simulink model "packetizer_core"  (R2016b)
settings: Solver=VariableStepAuto  StartTime=0.0  StopTime=2*64*512+100  RelTol=1e-3
model workspace (MAT data in the model file):
  dstin = [0 168430081 168430082 168430083 168430084 168430085 168430086 168430087 168430088 168430089 168430090 168430091 ... (33 elements, 1x33)]
  simin = [1 2 3 4 5 6 7 8 9 10 11 12 ... (262544 elements, 65636x4)]
libraries: xbsIndex_r4 x142
(part 2 of 2)

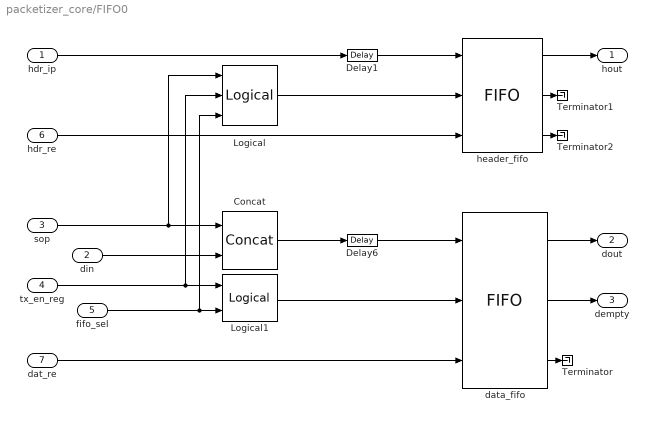
== system packetizer_core/FIFO0 ==
  hdr_ip : Inport
  din : Inport  Port=2
  sop : Inport  Port=3
  tx_en_reg : Inport  Port=4
  fifo_sel : Inport  Port=5
  hdr_re : Inport  Port=6
  dat_re : Inport  Port=7
  Concat : xbsIndex_r4/Concat  num_inputs=2  dbl_ovrd=off  block_type=concat
  Delay1 : xbsIndex_r4/Delay  rst=off  infoeditControl=Selection of Reset will increase slice count due to use of real FFs and instead of SRLs  en=off  latency=1  reg_retiming=off  dbl_ovrd=off  block_type=delay
  Delay6 : xbsIndex_r4/Delay  rst=off  infoeditControl=Selection of Reset will increase slice count due to use of real FFs and instead of SRLs  en=off  latency=1  reg_retiming=off  dbl_ovrd=off  block_type=delay
  Logical : xbsIndex_r4/Logical  logical_function=AND  inputs=3  en=off  latency=1  precision=Full  arith_type=Unsigned  n_bits=16  bin_pt=0  align_bp=on  dbl_ovrd=off  block_type=logical
  Logical1 : xbsIndex_r4/Logical  logical_function=AND  inputs=2  en=off  latency=1  precision=Full  arith_type=Unsigned  n_bits=16  bin_pt=0  align_bp=on  dbl_ovrd=off  block_type=logical
  Terminator : Terminator
  Terminator1 : Terminator
  Terminator2 : Terminator
  data_fifo : xbsIndex_r4/FIFO  mem_type=Block RAM  performance_options=First_Word_Fall_Through  embedded_registers=on  depth=16K  percent_nbits=1  rst=off  rst_latency=1  en=off  use_dcount=off  use_percent_full_port=off  use_almost_empty=off  almost_empty_thresh=2  use_almost_full=off  almost_full_thresh=14  explicit_period=off  dbl_ovrd=off  block_type=fifo
  header_fifo : xbsIndex_r4/FIFO  mem_type=Distributed RAM  performance_options=First_Word_Fall_Through  embedded_registers=off  depth=32  percent_nbits=1  rst=off  rst_latency=1  en=off  use_dcount=off  use_percent_full_port=off  use_almost_empty=off  almost_empty_thresh=2  use_almost_full=off  almost_full_thresh=14  explicit_period=off  dbl_ovrd=off  block_type=fifo
  hout : Outport
  dout : Outport  Port=2
  dempty : Outport  Port=3
  wires:
  Logical/1 -> header_fifo/2
  tx_en_reg/1 -> Logical1/1, Logical/2
  Delay1/1 -> header_fifo/1
  Delay6/1 -> data_fifo/1
  data_fifo/1 -> dout/1
  data_fifo/2 -> dempty/1
  Logical1/1 -> data_fifo/2
  dat_re/1 -> data_fifo/3
  hdr_re/1 -> header_fifo/3
  hdr_ip/1 -> Delay1/1
  Concat/1 -> Delay6/1
  header_fifo/1 -> hout/1
  sop/1 -> Concat/1, Logical/1
  din/1 -> Concat/2
  fifo_sel/1 -> Logical1/2, Logical/3
  data_fifo/3 -> Terminator/1
  header_fifo/2 -> Terminator1/1
  header_fifo/3 -> Terminator2/1

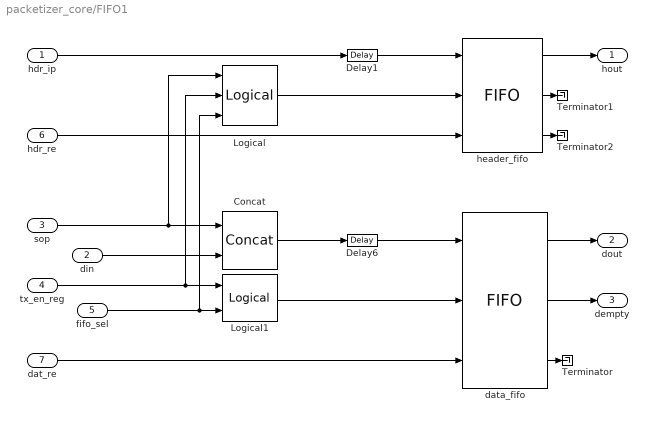
== system packetizer_core/FIFO1 ==
  hdr_ip : Inport
  din : Inport  Port=2
  sop : Inport  Port=3
  tx_en_reg : Inport  Port=4
  fifo_sel : Inport  Port=5
  hdr_re : Inport  Port=6
  dat_re : Inport  Port=7
  Concat : xbsIndex_r4/Concat  num_inputs=2  dbl_ovrd=off  block_type=concat
  Delay1 : xbsIndex_r4/Delay  rst=off  infoeditControl=Selection of Reset will increase slice count due to use of real FFs and instead of SRLs  en=off  latency=1  reg_retiming=off  dbl_ovrd=off  block_type=delay
  Delay6 : xbsIndex_r4/Delay  rst=off  infoeditControl=Selection of Reset will increase slice count due to use of real FFs and instead of SRLs  en=off  latency=1  reg_retiming=off  dbl_ovrd=off  block_type=delay
  Logical : xbsIndex_r4/Logical  logical_function=AND  inputs=3  en=off  latency=1  precision=Full  arith_type=Unsigned  n_bits=16  bin_pt=0  align_bp=on  dbl_ovrd=off  block_type=logical
  Logical1 : xbsIndex_r4/Logical  logical_function=AND  inputs=2  en=off  latency=1  precision=Full  arith_type=Unsigned  n_bits=16  bin_pt=0  align_bp=on  dbl_ovrd=off  block_type=logical
  Terminator : Terminator
  Terminator1 : Terminator
  Terminator2 : Terminator
  data_fifo : xbsIndex_r4/FIFO  mem_type=Block RAM  performance_options=First_Word_Fall_Through  embedded_registers=on  depth=16K  percent_nbits=1  rst=off  rst_latency=1  en=off  use_dcount=off  use_percent_full_port=off  use_almost_empty=off  almost_empty_thresh=2  use_almost_full=off  almost_full_thresh=14  explicit_period=off  dbl_ovrd=off  block_type=fifo
  header_fifo : xbsIndex_r4/FIFO  mem_type=Distributed RAM  performance_options=First_Word_Fall_Through  embedded_registers=off  depth=32  percent_nbits=1  rst=off  rst_latency=1  en=off  use_dcount=off  use_percent_full_port=off  use_almost_empty=off  almost_empty_thresh=2  use_almost_full=off  almost_full_thresh=14  explicit_period=off  dbl_ovrd=off  block_type=fifo
  hout : Outport
  dout : Outport  Port=2
  dempty : Outport  Port=3
  wires:
  Logical/1 -> header_fifo/2
  tx_en_reg/1 -> Logical1/1, Logical/2
  Delay1/1 -> header_fifo/1
  Delay6/1 -> data_fifo/1
  data_fifo/1 -> dout/1
  data_fifo/2 -> dempty/1
  Logical1/1 -> data_fifo/2
  dat_re/1 -> data_fifo/3
  hdr_re/1 -> header_fifo/3
  hdr_ip/1 -> Delay1/1
  Concat/1 -> Delay6/1
  header_fifo/1 -> hout/1
  sop/1 -> Concat/1, Logical/1
  din/1 -> Concat/2
  fifo_sel/1 -> Logical1/2, Logical/3
  data_fifo/3 -> Terminator/1
  header_fifo/2 -> Terminator1/1
  header_fifo/3 -> Terminator2/1

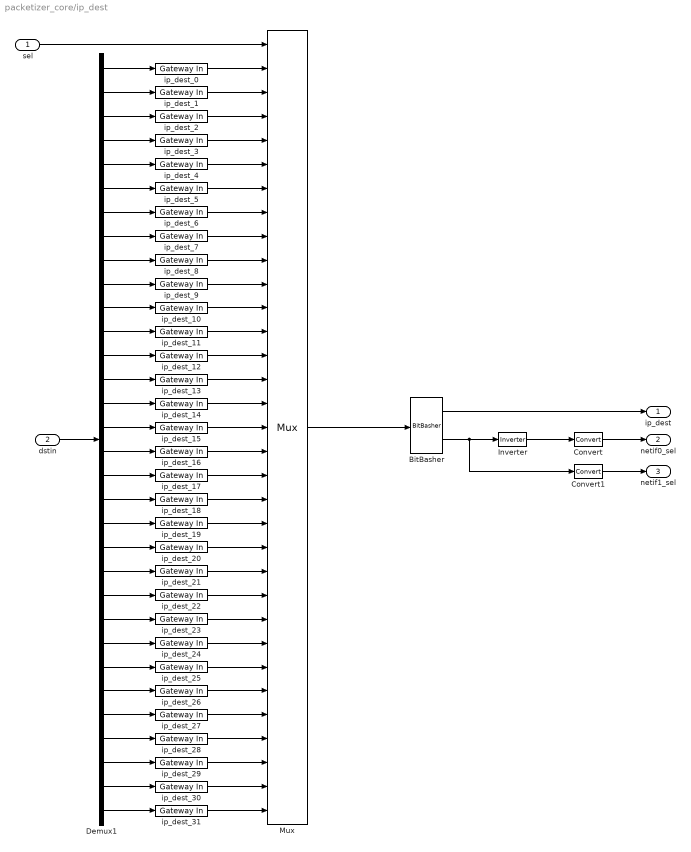
== system packetizer_core/ip_dest ==
  sel : Inport
  dstin : Inport  Port=2
  BitBasher : xbsIndex_r4/BitBasher  bitexpr=|  display_expr=off  sr_1=ip  arith_type1=Unsigned  bin_pt1=0  sr_2=sel  arith_type2=Unsigned  bin_pt2=0  sr_3=3  arith_type3=Unsigned  bin_pt3=0  sr_4=4  arith_type4=Unsigned  bin_pt4=0  dbl_ovrd=off  block_type=bitbasher
      | ip={in[31:25], 1'b0, in[23:0]}
      | sel={in[24]}
  Convert : xbsIndex_r4/Convert  gui_display_data_type=Boolean  arith_type=Boolean  n_bits=16  bin_pt=14  float_type=Single  exp_bits=8  fraction_bits=24  quantization=Truncate  overflow=Wrap  en=off  latency=0  pipeline=off  dbl_ovrd=off  block_type=convert
  Convert1 : xbsIndex_r4/Convert  gui_display_data_type=Boolean  arith_type=Boolean  n_bits=16  bin_pt=14  float_type=Single  exp_bits=8  fraction_bits=24  quantization=Truncate  overflow=Wrap  en=off  latency=0  pipeline=off  dbl_ovrd=off  block_type=convert
  Demux1 : Demux  Outputs=32
  Inverter : xbsIndex_r4/Inverter  en=off  latency=0  dbl_ovrd=off  block_type=inv
  Mux : xbsIndex_r4/Mux  inputs=32  en=off  latency=1  precision=Full  arith_type=Unsigned  n_bits=16  bin_pt=14  quantization=Truncate  overflow=Wrap  dbl_ovrd=off  block_type=mux
  ip_dest_{0..31} (32 alike) : xbsIndex_r4/Gateway In  gui_display_data_type=Fixed-point  arith_type=Unsigned  n_bits=32  bin_pt=0  preci_type=Single  exp_width=8  frac_width=24  rows=1  columns=1  quantization="Round  (unbiased: +/- Inf)"  overflow=Saturate  period=1  UseAsADC=off  ADCChannel='1'  interface=None  automatic_assignment=on  address_offset=hex2dec('00')  intf_name=''  intf_description=''  default_value=0  timing_constraint=None  locs_specified=off  LOCs={}  io_standard={}  inherit_from_input=off  hdl_port=on  dbl_ovrd=off  block_type=gatewayin
  ip_dest : Outport
  netif0_sel : Outport  Port=2
  netif1_sel : Outport  Port=3
  wires:
  ip_dest_6/1 -> Mux/8
  Demux1/16 -> ip_dest_15/1
  ip_dest_25/1 -> Mux/27
  Demux1/14 -> ip_dest_13/1
  ip_dest_3/1 -> Mux/5
  Demux1/26 -> ip_dest_25/1
  Demux1/18 -> ip_dest_17/1
  Demux1/32 -> ip_dest_31/1
  Demux1/4 -> ip_dest_3/1
  ip_dest_26/1 -> Mux/28
  ip_dest_23/1 -> Mux/25
  Demux1/10 -> ip_dest_9/1
  Demux1/7 -> ip_dest_6/1
  ip_dest_4/1 -> Mux/6
  ip_dest_8/1 -> Mux/10
  ip_dest_0/1 -> Mux/2
  ip_dest_13/1 -> Mux/15
  ip_dest_16/1 -> Mux/18
  ip_dest_12/1 -> Mux/14
  ip_dest_28/1 -> Mux/30
  ip_dest_7/1 -> Mux/9
  ip_dest_15/1 -> Mux/17
  Demux1/25 -> ip_dest_24/1
  Demux1/19 -> ip_dest_18/1
  Demux1/29 -> ip_dest_28/1
  ip_dest_2/1 -> Mux/4
  ip_dest_5/1 -> Mux/7
  Demux1/8 -> ip_dest_7/1
  Demux1/6 -> ip_dest_5/1
  Demux1/17 -> ip_dest_16/1
  Demux1/15 -> ip_dest_14/1
  Demux1/2 -> ip_dest_1/1
  ip_dest_11/1 -> Mux/13
  ip_dest_20/1 -> Mux/22
  ip_dest_1/1 -> Mux/3
  ip_dest_14/1 -> Mux/16
  Demux1/30 -> ip_dest_29/1
  Demux1/23 -> ip_dest_22/1
  Demux1/21 -> ip_dest_20/1
  Demux1/28 -> ip_dest_27/1
  ip_dest_21/1 -> Mux/23
  Demux1/27 -> ip_dest_26/1
  Demux1/11 -> ip_dest_10/1
  ip_dest_18/1 -> Mux/20
  ip_dest_10/1 -> Mux/12
  ip_dest_27/1 -> Mux/29
  Demux1/1 -> ip_dest_0/1
  Demux1/5 -> ip_dest_4/1
  Demux1/24 -> ip_dest_23/1
  ip_dest_30/1 -> Mux/32
  Demux1/3 -> ip_dest_2/1
  ip_dest_24/1 -> Mux/26
  Demux1/9 -> ip_dest_8/1
  sel/1 -> Mux/1
  dstin/1 -> Demux1/1
  Demux1/12 -> ip_dest_11/1
  ip_dest_17/1 -> Mux/19
  Demux1/20 -> ip_dest_19/1
  ip_dest_31/1 -> Mux/33
  Demux1/13 -> ip_dest_12/1
  ip_dest_19/1 -> Mux/21
  ip_dest_29/1 -> Mux/31
  ip_dest_22/1 -> Mux/24
  ip_dest_9/1 -> Mux/11
  Demux1/22 -> ip_dest_21/1
  Demux1/31 -> ip_dest_30/1
  Mux/1 -> BitBasher/1
  BitBasher/1 -> ip_dest/1
  BitBasher/2 -> Convert1/1, Inverter/1
  Inverter/1 -> Convert/1
  Convert/1 -> netif0_sel/1
  Convert1/1 -> netif1_sel/1

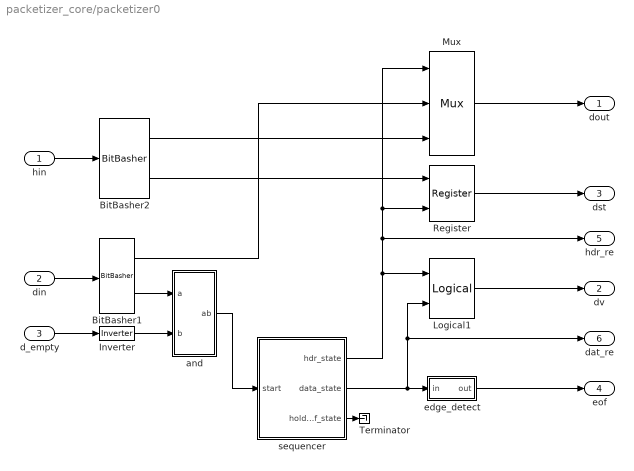
== system packetizer_core/packetizer0 ==
  hin : Inport
  din : Inport  Port=2
  d_empty : Inport  Port=3
  BitBasher1 : xbsIndex_r4/BitBasher  bitexpr=|  display_expr=off  sr_1=d  arith_type1=Unsigned  bin_pt1=0  sr_2=s  arith_type2=Unsigned  bin_pt2=0  sr_3=3  arith_type3=Unsigned  bin_pt3=0  sr_4=4  arith_type4=Unsigned  bin_pt4=0  dbl_ovrd=off  block_type=bitbasher
      | d={sd[63:0]}
      | s={sd[64]}
  BitBasher2 : xbsIndex_r4/BitBasher  bitexpr=|  display_expr=off  sr_1=hdr  arith_type1=Unsigned  bin_pt1=0  sr_2=ip  arith_type2=Unsigned  bin_pt2=0  sr_3=3  arith_type3=Unsigned  bin_pt3=0  sr_4=4  arith_type4=Unsigned  bin_pt4=0  dbl_ovrd=off  block_type=bitbasher
      | hdr={hdr_ip[95:32]}
      | ip={hdr_ip[31:0]}
  Inverter : xbsIndex_r4/Inverter  en=off  latency=0  dbl_ovrd=off  block_type=inv
  Logical1 : xbsIndex_r4/Logical  logical_function=OR  inputs=2  en=off  latency=1  precision=Full  arith_type=Unsigned  n_bits=16  bin_pt=0  align_bp=on  dbl_ovrd=off  block_type=logical
  Mux : xbsIndex_r4/Mux  inputs=2  en=off  latency=1  precision=Full  arith_type=Unsigned  n_bits=16  bin_pt=14  quantization=Truncate  overflow=Wrap  dbl_ovrd=off  block_type=mux
  Register : xbsIndex_r4/Register  init=0  rst=off  en=on  dbl_ovrd=off  block_type=register
  Terminator : Terminator
  and : Subsystem
  edge_detect : Subsystem  AncestorBlock=casper_library_misc/edge_detect  mask(edge_detect){edge=Falling, polarity=Active High, x_in=[0 0.08 0.08 0.16 0.16 0.24 0.24 0.32 0.32 0.4], y_in=[-1 -1  1  1  1  1  1  1  1  1], x_out=[0.6 0.68 0.68 0.76 0.76 0.84 0.84 0.92 0.92 1], y_out=[-1 -1  1  1 -1 -1 -1 -1 -1 -1]}
      mask prompts: edge "Edge Type"; polarity "Output Polarity"; x_in "Input X Positions"; y_in "Input Y Positions"; x_out "Output X Positions"; y_out "Output Y Positions"
      mask help: Output is active for one-cycle after each edge of the specified type (i.e. rising, falling or both).
      mask init:
      | edge_detect_init(gcb,...
      |     'edge',edge,...
      |     'polarity',polarity,...
      |     'x_in',x_in,...
      |     'x_out',x_out,...
      |     'y_in',y_in,...
      |     'y_out',y_out);
      | 
      | x_in_num=str2num(getfield(getfield(get_param(gcb,'UserData'),'parameters'),'x_in'));
      | x_out_num=str2num(getfield(getfield(get_param(gcb,'UserData'),'parameters'),'x_out'));
      | y_in_num=str2num(getfield(getfield(get_param(gcb,'UserData'),'parameters'),'y_in'));
      | y_out_num=str2num(getfield(getfield(get_param(gcb,'UserData'),'parameters'),'y_out'));
      settings: AttributesFormatString=|
      | falling edges
      | active high
      mask Help: Output is active for one-cycle after each edge of the specified type (i.e. rising, falling, or both).  Latency is zero.
      mask TypeOptions edge: Rising | Falling | Both
      mask TypeOptions polarity: Active High | Active Low
      mask Display:
      | plot(x_in_num,0.5+y_in_num*0.2);
      | plot(x_out_num,0.5+y_out_num*0.2);
  sequencer : Subsystem
  dout : Outport
  dv : Outport  Port=2
  dst : Outport  Port=3
  eof : Outport  Port=4
  hdr_re : Outport  Port=5
  dat_re : Outport  Port=6
  wires:
  din/1 -> BitBasher1/1
  d_empty/1 -> Inverter/1
  sequencer/1(hdr_state) -> Register/2, Mux/1, hdr_re/1, Logical1/1
  BitBasher1/1 -> Mux/2
  Mux/1 -> dout/1
  hin/1 -> BitBasher2/1
  BitBasher2/1 -> Mux/3
  Register/1 -> dst/1
  BitBasher2/2 -> Register/1
  sequencer/2(data_state) -> dat_re/1, Logical1/2, edge_detect/1(in)
  edge_detect/1(out) -> eof/1
  Logical1/1 -> dv/1
  sequencer/3(holdoff_state) -> Terminator/1
  BitBasher1/2 -> and/1(a)
  Inverter/1 -> and/2(b)
  and/1(ab) -> sequencer/1(start)

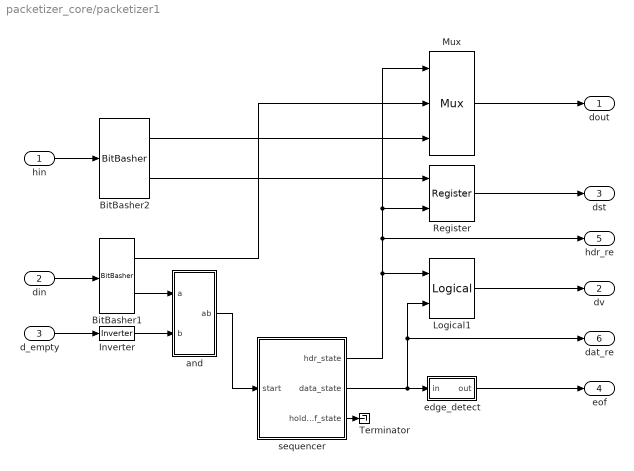
== system packetizer_core/packetizer1 ==
  hin : Inport
  din : Inport  Port=2
  d_empty : Inport  Port=3
  BitBasher1 : xbsIndex_r4/BitBasher  bitexpr=|  display_expr=off  sr_1=d  arith_type1=Unsigned  bin_pt1=0  sr_2=s  arith_type2=Unsigned  bin_pt2=0  sr_3=3  arith_type3=Unsigned  bin_pt3=0  sr_4=4  arith_type4=Unsigned  bin_pt4=0  dbl_ovrd=off  block_type=bitbasher
      | d={sd[63:0]}
      | s={sd[64]}
  BitBasher2 : xbsIndex_r4/BitBasher  bitexpr=|  display_expr=off  sr_1=hdr  arith_type1=Unsigned  bin_pt1=0  sr_2=ip  arith_type2=Unsigned  bin_pt2=0  sr_3=3  arith_type3=Unsigned  bin_pt3=0  sr_4=4  arith_type4=Unsigned  bin_pt4=0  dbl_ovrd=off  block_type=bitbasher
      | hdr={hdr_ip[95:32]}
      | ip={hdr_ip[31:0]}
  Inverter : xbsIndex_r4/Inverter  en=off  latency=0  dbl_ovrd=off  block_type=inv
  Logical1 : xbsIndex_r4/Logical  logical_function=OR  inputs=2  en=off  latency=1  precision=Full  arith_type=Unsigned  n_bits=16  bin_pt=0  align_bp=on  dbl_ovrd=off  block_type=logical
  Mux : xbsIndex_r4/Mux  inputs=2  en=off  latency=1  precision=Full  arith_type=Unsigned  n_bits=16  bin_pt=14  quantization=Truncate  overflow=Wrap  dbl_ovrd=off  block_type=mux
  Register : xbsIndex_r4/Register  init=0  rst=off  en=on  dbl_ovrd=off  block_type=register
  Terminator : Terminator
  and : Subsystem
  edge_detect : Subsystem  AncestorBlock=casper_library_misc/edge_detect  mask(edge_detect){edge=Falling, polarity=Active High, x_in=[0 0.08 0.08 0.16 0.16 0.24 0.24 0.32 0.32 0.4], y_in=[-1 -1  1  1  1  1  1  1  1  1], x_out=[0.6 0.68 0.68 0.76 0.76 0.84 0.84 0.92 0.92 1], y_out=[-1 -1  1  1 -1 -1 -1 -1 -1 -1]}
      mask prompts: edge "Edge Type"; polarity "Output Polarity"; x_in "Input X Positions"; y_in "Input Y Positions"; x_out "Output X Positions"; y_out "Output Y Positions"
      mask help: Output is active for one-cycle after each edge of the specified type (i.e. rising, falling or both).
      mask init: same as packetizer_core/packetizer0/edge_detect
      settings: AttributesFormatString=|
      | falling edges
      | active high
      mask Help: Output is active for one-cycle after each edge of the specified type (i.e. rising, falling, or both).  Latency is zero.
      mask TypeOptions edge: Rising | Falling | Both
      mask TypeOptions polarity: Active High | Active Low
      mask Display:
      | plot(x_in_num,0.5+y_in_num*0.2);
      | plot(x_out_num,0.5+y_out_num*0.2);
  sequencer : Subsystem
  dout : Outport
  dv : Outport  Port=2
  dst : Outport  Port=3
  eof : Outport  Port=4
  hdr_re : Outport  Port=5
  dat_re : Outport  Port=6
  wires:
  din/1 -> BitBasher1/1
  d_empty/1 -> Inverter/1
  sequencer/1(hdr_state) -> Register/2, Mux/1, hdr_re/1, Logical1/1
  BitBasher1/1 -> Mux/2
  Mux/1 -> dout/1
  hin/1 -> BitBasher2/1
  BitBasher2/1 -> Mux/3
  Register/1 -> dst/1
  BitBasher2/2 -> Register/1
  sequencer/2(data_state) -> dat_re/1, Logical1/2, edge_detect/1(in)
  edge_detect/1(out) -> eof/1
  Logical1/1 -> dv/1
  sequencer/3(holdoff_state) -> Terminator/1
  BitBasher1/2 -> and/1(a)
  Inverter/1 -> and/2(b)
  and/1(ab) -> sequencer/1(start)

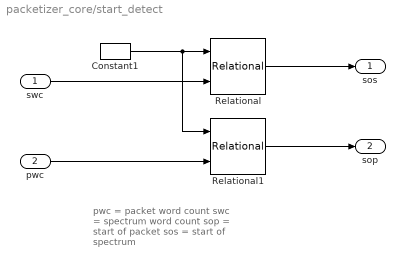
== system packetizer_core/start_detect ==
  note: pwc = packet word count
      | swc = spectrum word count
      |
      | sop = start of packet
      | sos = start of spectrum
  swc : Inport
  pwc : Inport  Port=2
  Constant1 : xbsIndex_r4/Constant  const=0  gui_display_data_type=Fixed-point  arith_type=Signed (2's comp)  n_bits=1  bin_pt=0  preci_type=Single  exp_width=8  frac_width=24  explicit_period=on  period=1  equ=P=C  opselect=C  inp2=PCIN>>17  opr=+  inp1=P  carry=CIN  dbl_ovrd=off  block_type=constant
  Relational : xbsIndex_r4/Relational  mode=a=b  op_type=Bool  en=off  latency=1  dbl_ovrd=off  block_type=relational
  Relational1 : xbsIndex_r4/Relational  mode=a=b  op_type=Bool  en=off  latency=1  dbl_ovrd=off  block_type=relational
  sos : Outport
  sop : Outport  Port=2
  wires:
  pwc/1 -> Relational1/2
  Relational1/1 -> sop/1
  Constant1/1 -> Relational1/1, Relational/1
  Relational/1 -> sos/1
  swc/1 -> Relational/2

== system packetizer_core/packetizer0/and ==
  a : Inport
  b : Inport  Port=2
  Convert : xbsIndex_r4/Convert  gui_display_data_type=Boolean  arith_type=Boolean  n_bits=16  bin_pt=14  float_type=Single  exp_bits=8  fraction_bits=24  quantization=Truncate  overflow=Wrap  en=off  latency=0  pipeline=off  dbl_ovrd=off  block_type=convert
  Logical : xbsIndex_r4/Logical  logical_function=AND  inputs=2  en=off  latency=0  precision=Full  arith_type=Unsigned  n_bits=16  bin_pt=0  align_bp=on  dbl_ovrd=off  block_type=logical
  ab : Outport
  wires:
  Logical/1 -> ab/1
  a/1 -> Convert/1
  b/1 -> Logical/2
  Convert/1 -> Logical/1

== system packetizer_core/packetizer0/edge_detect ==
  in : Inport
  Delay : xbsIndex_r4/Delay  rst=off  infoeditControl=Selection of Reset will increase slice count due to use of real FFs and instead of SRLs  en=off  latency=1  reg_retiming=off  dbl_ovrd=off  block_type=delay
      settings: xl_area=[0, 0, 0, 0, 0, 0, 0]
  Inverter : xbsIndex_r4/Inverter  en=off  latency=0  dbl_ovrd=off  block_type=inv
      settings: xl_area=[0, 0, 0, 0, 0, 0, 0]
  edge_op : xbsIndex_r4/Logical  logical_function=AND  inputs=2  en=off  latency=0  precision=Full  arith_type=Unsigned  n_bits=8  bin_pt=2  align_bp=on  dbl_ovrd=off  block_type=logical
      settings: xl_area=[0, 0, 0, 0, 0, 0, 0]
  out : Outport
  wires:
  Inverter/1 -> edge_op/1
  edge_op/1 -> out/1
  in/1 -> Inverter/1, Delay/1
  Delay/1 -> edge_op/2

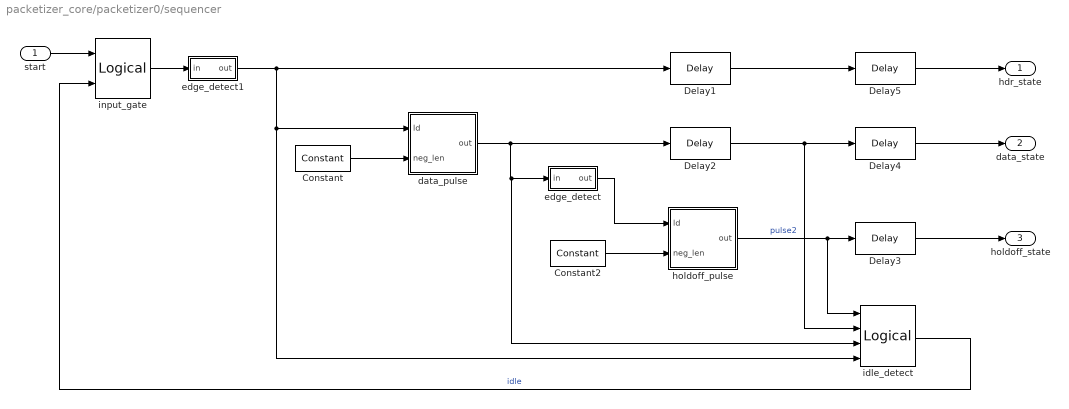
== system packetizer_core/packetizer0/sequencer ==
  start : Inport
  Constant : xbsIndex_r4/Constant  const=-1024  gui_display_data_type=Fixed-point  arith_type=Signed (2's comp)  n_bits=11  bin_pt=0  preci_type=Single  exp_width=8  frac_width=24  explicit_period=off  period=1  equ=P=C  opselect=C  inp2=PCIN>>17  opr=+  inp1=P  carry=CIN  dbl_ovrd=off  block_type=constant
  Constant2 : xbsIndex_r4/Constant  const=-(445-2)  gui_display_data_type=Fixed-point  arith_type=Signed (2's comp)  n_bits=11  bin_pt=0  preci_type=Single  exp_width=8  frac_width=24  explicit_period=off  period=1  equ=P=C  opselect=C  inp2=PCIN>>17  opr=+  inp1=P  carry=CIN  dbl_ovrd=off  block_type=constant
  Delay{1..5} (5 alike) : xbsIndex_r4/Delay  rst=off  infoeditControl=Selection of Reset will increase slice count due to use of real FFs and instead of SRLs  en=off  latency=1  reg_retiming=off  dbl_ovrd=off  block_type=delay
  data_pulse : Subsystem
  edge_detect : Subsystem  AncestorBlock=casper_library_misc/edge_detect  mask(edge_detect){edge=Falling, polarity=Active High, x_in=[0 0.08 0.08 0.16 0.16 0.24 0.24 0.32 0.32 0.4], y_in=[-1 -1  1  1  1  1  1  1  1  1], x_out=[0.6 0.68 0.68 0.76 0.76 0.84 0.84 0.92 0.92 1], y_out=[-1 -1  1  1 -1 -1 -1 -1 -1 -1]}
      mask prompts: edge "Edge Type"; polarity "Output Polarity"; x_in "Input X Positions"; y_in "Input Y Positions"; x_out "Output X Positions"; y_out "Output Y Positions"
      mask help: Output is active for one-cycle after each edge of the specified type (i.e. rising, falling or both).
      mask init: same as packetizer_core/packetizer0/edge_detect
      settings: AttributesFormatString=|
      | falling edges
      | active high
      mask Help: Output is active for one-cycle after each edge of the specified type (i.e. rising, falling, or both).  Latency is zero.
      mask TypeOptions edge: Rising | Falling | Both
      mask TypeOptions polarity: Active High | Active Low
      mask Display:
      | plot(x_in_num,0.5+y_in_num*0.2);
      | plot(x_out_num,0.5+y_out_num*0.2);
  edge_detect1 : Subsystem  AncestorBlock=casper_library_misc/edge_detect  mask(edge_detect){edge=Rising, polarity=Active High, x_in=[0 0.08 0.08 0.16 0.16 0.24 0.24 0.32 0.32 0.4], y_in=[-1 -1  1  1  1  1  1  1  1  1], x_out=[0.6 0.68 0.68 0.76 0.76 0.84 0.84 0.92 0.92 1], y_out=[-1 -1  1  1 -1 -1 -1 -1 -1 -1]}
      mask prompts: edge "Edge Type"; polarity "Output Polarity"; x_in "Input X Positions"; y_in "Input Y Positions"; x_out "Output X Positions"; y_out "Output Y Positions"
      mask help: Output is active for one-cycle after each edge of the specified type (i.e. rising, falling or both).
      mask init: same as packetizer_core/packetizer0/edge_detect
      settings: AttributesFormatString=|
      | rising edges
      | active high
      mask Help: Output is active for one-cycle after each edge of the specified type (i.e. rising, falling, or both).  Latency is zero.
      mask TypeOptions edge: Rising | Falling | Both
      mask TypeOptions polarity: Active High | Active Low
      mask Display:
      | plot(x_in_num,0.5+y_in_num*0.2);
      | plot(x_out_num,0.5+y_out_num*0.2);
  holdoff_pulse : Subsystem
  idle_detect : xbsIndex_r4/Logical  logical_function=NOR  inputs=4  en=off  latency=1  precision=Full  arith_type=Unsigned  n_bits=16  bin_pt=0  align_bp=on  dbl_ovrd=off  block_type=logical
  input_gate : xbsIndex_r4/Logical  logical_function=AND  inputs=2  en=off  latency=0  precision=Full  arith_type=Unsigned  n_bits=16  bin_pt=0  align_bp=on  dbl_ovrd=off  block_type=logical
  hdr_state : Outport
  data_state : Outport  Port=2
  holdoff_state : Outport  Port=3
  wires:
  Delay5/1 -> hdr_state/1
  edge_detect/1(out) -> holdoff_pulse/1(ld)
  holdoff_pulse/1(out) -> idle_detect/1, Delay3/1  "pulse2"
  edge_detect1/1(out) -> Delay1/1, idle_detect/4, data_pulse/1(ld)
  Constant/1 -> data_pulse/2(neg_len)
  Delay4/1 -> data_state/1
  Delay1/1 -> Delay5/1
  Delay3/1 -> holdoff_state/1
  data_pulse/1(out) -> Delay2/1, idle_detect/3, edge_detect/1(in)
  Delay2/1 -> idle_detect/2, Delay4/1
  Constant2/1 -> holdoff_pulse/2(neg_len)
  input_gate/1 -> edge_detect1/1(in)
  start/1 -> input_gate/1
  idle_detect/1 -> input_gate/2  "idle"

== system packetizer_core/packetizer1/and ==
  a : Inport
  b : Inport  Port=2
  Convert : xbsIndex_r4/Convert  gui_display_data_type=Boolean  arith_type=Boolean  n_bits=16  bin_pt=14  float_type=Single  exp_bits=8  fraction_bits=24  quantization=Truncate  overflow=Wrap  en=off  latency=0  pipeline=off  dbl_ovrd=off  block_type=convert
  Logical : xbsIndex_r4/Logical  logical_function=AND  inputs=2  en=off  latency=0  precision=Full  arith_type=Unsigned  n_bits=16  bin_pt=0  align_bp=on  dbl_ovrd=off  block_type=logical
  ab : Outport
  wires:
  Logical/1 -> ab/1
  a/1 -> Convert/1
  b/1 -> Logical/2
  Convert/1 -> Logical/1

== system packetizer_core/packetizer1/edge_detect ==
  in : Inport
  Delay : xbsIndex_r4/Delay  rst=off  infoeditControl=Selection of Reset will increase slice count due to use of real FFs and instead of SRLs  en=off  latency=1  reg_retiming=off  dbl_ovrd=off  block_type=delay
      settings: xl_area=[0, 0, 0, 0, 0, 0, 0]
  Inverter : xbsIndex_r4/Inverter  en=off  latency=0  dbl_ovrd=off  block_type=inv
      settings: xl_area=[0, 0, 0, 0, 0, 0, 0]
  edge_op : xbsIndex_r4/Logical  logical_function=AND  inputs=2  en=off  latency=0  precision=Full  arith_type=Unsigned  n_bits=8  bin_pt=2  align_bp=on  dbl_ovrd=off  block_type=logical
      settings: xl_area=[0, 0, 0, 0, 0, 0, 0]
  out : Outport
  wires:
  Inverter/1 -> edge_op/1
  edge_op/1 -> out/1
  in/1 -> Inverter/1, Delay/1
  Delay/1 -> edge_op/2

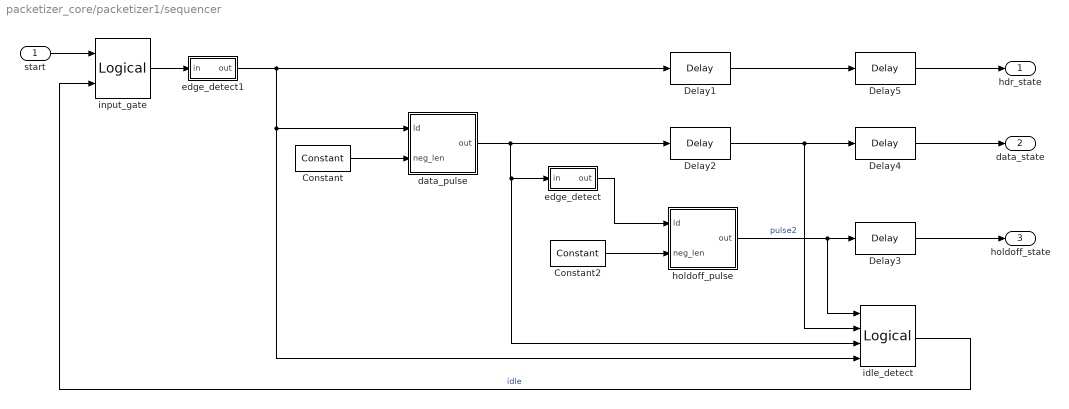
== system packetizer_core/packetizer1/sequencer ==
  start : Inport
  Constant : xbsIndex_r4/Constant  const=-1024  gui_display_data_type=Fixed-point  arith_type=Signed (2's comp)  n_bits=11  bin_pt=0  preci_type=Single  exp_width=8  frac_width=24  explicit_period=off  period=1  equ=P=C  opselect=C  inp2=PCIN>>17  opr=+  inp1=P  carry=CIN  dbl_ovrd=off  block_type=constant
  Constant2 : xbsIndex_r4/Constant  const=-(445-2)  gui_display_data_type=Fixed-point  arith_type=Signed (2's comp)  n_bits=11  bin_pt=0  preci_type=Single  exp_width=8  frac_width=24  explicit_period=off  period=1  equ=P=C  opselect=C  inp2=PCIN>>17  opr=+  inp1=P  carry=CIN  dbl_ovrd=off  block_type=constant
  Delay{1..5} (5 alike) : xbsIndex_r4/Delay  rst=off  infoeditControl=Selection of Reset will increase slice count due to use of real FFs and instead of SRLs  en=off  latency=1  reg_retiming=off  dbl_ovrd=off  block_type=delay
  data_pulse : Subsystem
  edge_detect : Subsystem  AncestorBlock=casper_library_misc/edge_detect  mask(edge_detect){edge=Falling, polarity=Active High, x_in=[0 0.08 0.08 0.16 0.16 0.24 0.24 0.32 0.32 0.4], y_in=[-1 -1  1  1  1  1  1  1  1  1], x_out=[0.6 0.68 0.68 0.76 0.76 0.84 0.84 0.92 0.92 1], y_out=[-1 -1  1  1 -1 -1 -1 -1 -1 -1]}
      mask prompts: edge "Edge Type"; polarity "Output Polarity"; x_in "Input X Positions"; y_in "Input Y Positions"; x_out "Output X Positions"; y_out "Output Y Positions"
      mask help: Output is active for one-cycle after each edge of the specified type (i.e. rising, falling or both).
      mask init: same as packetizer_core/packetizer0/edge_detect
      settings: AttributesFormatString=|
      | falling edges
      | active high
      mask Help: Output is active for one-cycle after each edge of the specified type (i.e. rising, falling, or both).  Latency is zero.
      mask TypeOptions edge: Rising | Falling | Both
      mask TypeOptions polarity: Active High | Active Low
      mask Display:
      | plot(x_in_num,0.5+y_in_num*0.2);
      | plot(x_out_num,0.5+y_out_num*0.2);
  edge_detect1 : Subsystem  AncestorBlock=casper_library_misc/edge_detect  mask(edge_detect){edge=Rising, polarity=Active High, x_in=[0 0.08 0.08 0.16 0.16 0.24 0.24 0.32 0.32 0.4], y_in=[-1 -1  1  1  1  1  1  1  1  1], x_out=[0.6 0.68 0.68 0.76 0.76 0.84 0.84 0.92 0.92 1], y_out=[-1 -1  1  1 -1 -1 -1 -1 -1 -1]}
      mask prompts: edge "Edge Type"; polarity "Output Polarity"; x_in "Input X Positions"; y_in "Input Y Positions"; x_out "Output X Positions"; y_out "Output Y Positions"
      mask help: Output is active for one-cycle after each edge of the specified type (i.e. rising, falling or both).
      mask init: same as packetizer_core/packetizer0/edge_detect
      settings: AttributesFormatString=|
      | rising edges
      | active high
      mask Help: Output is active for one-cycle after each edge of the specified type (i.e. rising, falling, or both).  Latency is zero.
      mask TypeOptions edge: Rising | Falling | Both
      mask TypeOptions polarity: Active High | Active Low
      mask Display:
      | plot(x_in_num,0.5+y_in_num*0.2);
      | plot(x_out_num,0.5+y_out_num*0.2);
  holdoff_pulse : Subsystem
  idle_detect : xbsIndex_r4/Logical  logical_function=NOR  inputs=4  en=off  latency=1  precision=Full  arith_type=Unsigned  n_bits=16  bin_pt=0  align_bp=on  dbl_ovrd=off  block_type=logical
  input_gate : xbsIndex_r4/Logical  logical_function=AND  inputs=2  en=off  latency=0  precision=Full  arith_type=Unsigned  n_bits=16  bin_pt=0  align_bp=on  dbl_ovrd=off  block_type=logical
  hdr_state : Outport
  data_state : Outport  Port=2
  holdoff_state : Outport  Port=3
  wires:
  Delay5/1 -> hdr_state/1
  edge_detect/1(out) -> holdoff_pulse/1(ld)
  holdoff_pulse/1(out) -> idle_detect/1, Delay3/1  "pulse2"
  edge_detect1/1(out) -> Delay1/1, idle_detect/4, data_pulse/1(ld)
  Constant/1 -> data_pulse/2(neg_len)
  Delay4/1 -> data_state/1
  Delay1/1 -> Delay5/1
  Delay3/1 -> holdoff_state/1
  data_pulse/1(out) -> Delay2/1, idle_detect/3, edge_detect/1(in)
  Delay2/1 -> idle_detect/2, Delay4/1
  Constant2/1 -> holdoff_pulse/2(neg_len)
  input_gate/1 -> edge_detect1/1(in)
  start/1 -> input_gate/1
  idle_detect/1 -> input_gate/2  "idle"

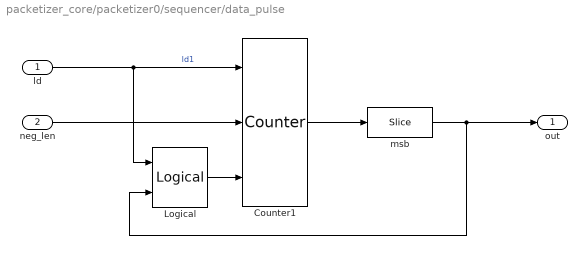
== system packetizer_core/packetizer0/sequencer/data_pulse ==
  ld : Inport
  neg_len : Inport  Port=2
  Counter1 : xbsIndex_r4/Counter  cnt_type=Free Running  cnt_to=Inf  operation=Up  start_count=0  cnt_by_val=1  arith_type="Signed  (2's comp)"  n_bits=11  bin_pt=0  load_pin=on  rst=off  en=on  explicit_period=on  period=1  use_behavioral_HDL=off  implementation=Fabric  dbl_ovrd=off  block_type=counter
  Logical : xbsIndex_r4/Logical  logical_function=OR  inputs=2  en=off  latency=0  precision=Full  arith_type=Unsigned  n_bits=16  bin_pt=0  align_bp=on  dbl_ovrd=off  block_type=logical
  msb : xbsIndex_r4/Slice  nbits=1  boolean_output=on  mode=Upper Bit Location + Width  bit1=0  base1=MSB of Input  bit0=0  base0=LSB of Input  dbl_ovrd=off  block_type=slice
  out : Outport
  wires:
  Logical/1 -> Counter1/3
  Counter1/1 -> msb/1
  ld/1 -> Logical/1, Counter1/1  "ld1"
  msb/1 -> out/1, Logical/2
  neg_len/1 -> Counter1/2

== system packetizer_core/packetizer0/sequencer/edge_detect ==
  in : Inport
  Delay : xbsIndex_r4/Delay  rst=off  infoeditControl=Selection of Reset will increase slice count due to use of real FFs and instead of SRLs  en=off  latency=1  reg_retiming=off  dbl_ovrd=off  block_type=delay
      settings: xl_area=[0, 0, 0, 0, 0, 0, 0]
  Inverter : xbsIndex_r4/Inverter  en=off  latency=0  dbl_ovrd=off  block_type=inv
      settings: xl_area=[0, 0, 0, 0, 0, 0, 0]
  edge_op : xbsIndex_r4/Logical  logical_function=AND  inputs=2  en=off  latency=0  precision=Full  arith_type=Unsigned  n_bits=8  bin_pt=2  align_bp=on  dbl_ovrd=off  block_type=logical
      settings: xl_area=[0, 0, 0, 0, 0, 0, 0]
  out : Outport
  wires:
  Inverter/1 -> edge_op/1
  edge_op/1 -> out/1
  in/1 -> Inverter/1, Delay/1
  Delay/1 -> edge_op/2

== system packetizer_core/packetizer0/sequencer/edge_detect1 ==
  in : Inport
  Delay : xbsIndex_r4/Delay  rst=off  infoeditControl=Selection of Reset will increase slice count due to use of real FFs and instead of SRLs  en=off  latency=1  reg_retiming=off  dbl_ovrd=off  block_type=delay
      settings: xl_area=[0, 0, 0, 0, 0, 0, 0]
  Inverter : xbsIndex_r4/Inverter  en=off  latency=0  dbl_ovrd=off  block_type=inv
      settings: xl_area=[0, 0, 0, 0, 0, 0, 0]
  edge_op : xbsIndex_r4/Logical  logical_function=NOR  inputs=2  en=off  latency=0  precision=Full  arith_type=Unsigned  n_bits=8  bin_pt=2  align_bp=on  dbl_ovrd=off  block_type=logical
      settings: xl_area=[0, 0, 0, 0, 0, 0, 0]
  out : Outport
  wires:
  Inverter/1 -> edge_op/1
  edge_op/1 -> out/1
  in/1 -> Inverter/1, Delay/1
  Delay/1 -> edge_op/2

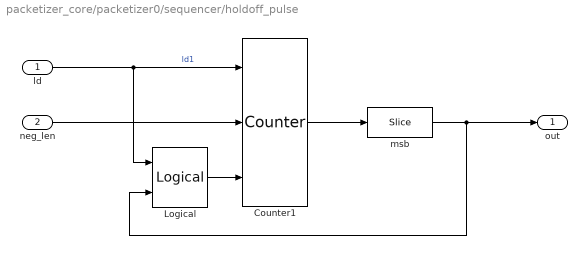
== system packetizer_core/packetizer0/sequencer/holdoff_pulse ==
  ld : Inport
  neg_len : Inport  Port=2
  Counter1 : xbsIndex_r4/Counter  cnt_type=Free Running  cnt_to=Inf  operation=Up  start_count=0  cnt_by_val=1  arith_type="Signed  (2's comp)"  n_bits=11  bin_pt=0  load_pin=on  rst=off  en=on  explicit_period=on  period=1  use_behavioral_HDL=off  implementation=Fabric  dbl_ovrd=off  block_type=counter
  Logical : xbsIndex_r4/Logical  logical_function=OR  inputs=2  en=off  latency=0  precision=Full  arith_type=Unsigned  n_bits=16  bin_pt=0  align_bp=on  dbl_ovrd=off  block_type=logical
  msb : xbsIndex_r4/Slice  nbits=1  boolean_output=on  mode=Upper Bit Location + Width  bit1=0  base1=MSB of Input  bit0=0  base0=LSB of Input  dbl_ovrd=off  block_type=slice
  out : Outport
  wires:
  Logical/1 -> Counter1/3
  Counter1/1 -> msb/1
  ld/1 -> Logical/1, Counter1/1  "ld1"
  msb/1 -> out/1, Logical/2
  neg_len/1 -> Counter1/2

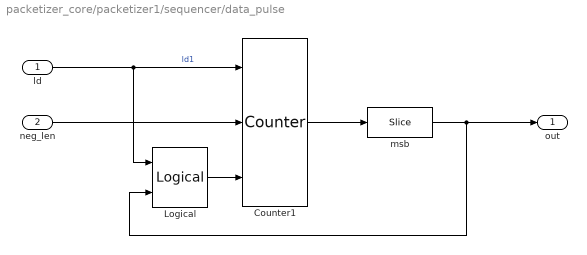
== system packetizer_core/packetizer1/sequencer/data_pulse ==
  ld : Inport
  neg_len : Inport  Port=2
  Counter1 : xbsIndex_r4/Counter  cnt_type=Free Running  cnt_to=Inf  operation=Up  start_count=0  cnt_by_val=1  arith_type="Signed  (2's comp)"  n_bits=11  bin_pt=0  load_pin=on  rst=off  en=on  explicit_period=on  period=1  use_behavioral_HDL=off  implementation=Fabric  dbl_ovrd=off  block_type=counter
  Logical : xbsIndex_r4/Logical  logical_function=OR  inputs=2  en=off  latency=0  precision=Full  arith_type=Unsigned  n_bits=16  bin_pt=0  align_bp=on  dbl_ovrd=off  block_type=logical
  msb : xbsIndex_r4/Slice  nbits=1  boolean_output=on  mode=Upper Bit Location + Width  bit1=0  base1=MSB of Input  bit0=0  base0=LSB of Input  dbl_ovrd=off  block_type=slice
  out : Outport
  wires:
  Logical/1 -> Counter1/3
  Counter1/1 -> msb/1
  ld/1 -> Logical/1, Counter1/1  "ld1"
  msb/1 -> out/1, Logical/2
  neg_len/1 -> Counter1/2

== system packetizer_core/packetizer1/sequencer/edge_detect ==
  in : Inport
  Delay : xbsIndex_r4/Delay  rst=off  infoeditControl=Selection of Reset will increase slice count due to use of real FFs and instead of SRLs  en=off  latency=1  reg_retiming=off  dbl_ovrd=off  block_type=delay
      settings: xl_area=[0, 0, 0, 0, 0, 0, 0]
  Inverter : xbsIndex_r4/Inverter  en=off  latency=0  dbl_ovrd=off  block_type=inv
      settings: xl_area=[0, 0, 0, 0, 0, 0, 0]
  edge_op : xbsIndex_r4/Logical  logical_function=AND  inputs=2  en=off  latency=0  precision=Full  arith_type=Unsigned  n_bits=8  bin_pt=2  align_bp=on  dbl_ovrd=off  block_type=logical
      settings: xl_area=[0, 0, 0, 0, 0, 0, 0]
  out : Outport
  wires:
  Inverter/1 -> edge_op/1
  edge_op/1 -> out/1
  in/1 -> Inverter/1, Delay/1
  Delay/1 -> edge_op/2

== system packetizer_core/packetizer1/sequencer/edge_detect1 ==
  in : Inport
  Delay : xbsIndex_r4/Delay  rst=off  infoeditControl=Selection of Reset will increase slice count due to use of real FFs and instead of SRLs  en=off  latency=1  reg_retiming=off  dbl_ovrd=off  block_type=delay
      settings: xl_area=[0, 0, 0, 0, 0, 0, 0]
  Inverter : xbsIndex_r4/Inverter  en=off  latency=0  dbl_ovrd=off  block_type=inv
      settings: xl_area=[0, 0, 0, 0, 0, 0, 0]
  edge_op : xbsIndex_r4/Logical  logical_function=NOR  inputs=2  en=off  latency=0  precision=Full  arith_type=Unsigned  n_bits=8  bin_pt=2  align_bp=on  dbl_ovrd=off  block_type=logical
      settings: xl_area=[0, 0, 0, 0, 0, 0, 0]
  out : Outport
  wires:
  Inverter/1 -> edge_op/1
  edge_op/1 -> out/1
  in/1 -> Inverter/1, Delay/1
  Delay/1 -> edge_op/2

== system packetizer_core/packetizer1/sequencer/holdoff_pulse ==
  ld : Inport
  neg_len : Inport  Port=2
  Counter1 : xbsIndex_r4/Counter  cnt_type=Free Running  cnt_to=Inf  operation=Up  start_count=0  cnt_by_val=1  arith_type="Signed  (2's comp)"  n_bits=11  bin_pt=0  load_pin=on  rst=off  en=on  explicit_period=on  period=1  use_behavioral_HDL=off  implementation=Fabric  dbl_ovrd=off  block_type=counter
  Logical : xbsIndex_r4/Logical  logical_function=OR  inputs=2  en=off  latency=0  precision=Full  arith_type=Unsigned  n_bits=16  bin_pt=0  align_bp=on  dbl_ovrd=off  block_type=logical
  msb : xbsIndex_r4/Slice  nbits=1  boolean_output=on  mode=Upper Bit Location + Width  bit1=0  base1=MSB of Input  bit0=0  base0=LSB of Input  dbl_ovrd=off  block_type=slice
  out : Outport
  wires:
  Logical/1 -> Counter1/3
  Counter1/1 -> msb/1
  ld/1 -> Logical/1, Counter1/1  "ld1"
  msb/1 -> out/1, Logical/2
  neg_len/1 -> Counter1/2
